simulink model "Grading_system"  (R2021a)
settings: Solver=VariableStepAuto  StartTime=0.0  StopTime=10.0  RelTol=1e-3
settings Model: Creator=Nour  LastModifiedBy=Nour

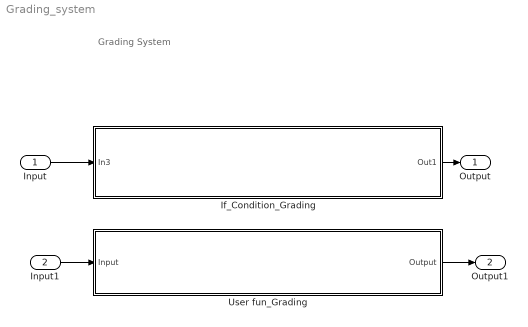
== system Grading_system ==
  note: Grading System
  Input : Inport
  Input1 : Inport  Port=2  OutDataTypeStr=uint8
  If_Condition_Grading : Subsystem
  User fun_Grading : Subsystem
  Output : Outport
  Output1 : Outport  Port=2
  wires:
  Input/1 -> If_Condition_Grading/1(In3)
  If_Condition_Grading/1(Out1) -> Output/1
  User fun_Grading/1(Output) -> Output1/1
  Input1/1 -> User fun_Grading/1(Input)

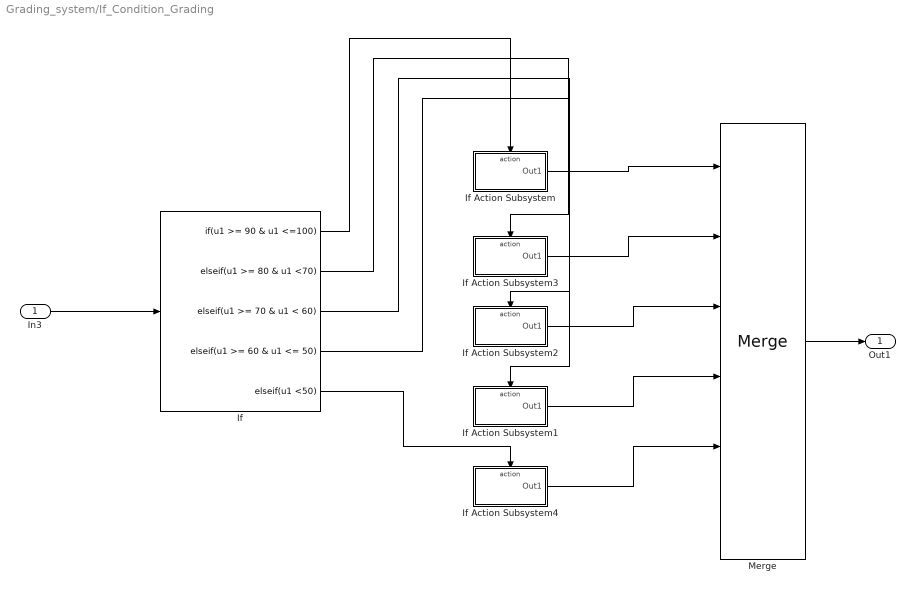
== system Grading_system/If_Condition_Grading ==
  In3 : Inport  OutDataTypeStr=uint8
  If : If  IfExpression=u1 >= 90 & u1 <=100  ElseIfExpressions=u1 >= 80 & u1 <70 , u1 >= 70 & u1 < 60, u1 >= 60 & u1 <= 50,u1 <50  ShowElse=off
  If Action Subsystem : Subsystem  TreatAsAtomicUnit=on
  If Action Subsystem1 : Subsystem  TreatAsAtomicUnit=on
  If Action Subsystem2 : Subsystem  TreatAsAtomicUnit=on
  If Action Subsystem3 : Subsystem  TreatAsAtomicUnit=on
  If Action Subsystem4 : Subsystem  TreatAsAtomicUnit=on
  Merge : Merge  Inputs=6
  Out1 : Outport
  wires:
  If Action Subsystem1/1(Out1) -> Merge/4
  If/4 -> If Action Subsystem1/Action
  If/3 -> If Action Subsystem2/Action
  If Action Subsystem4/1(Out1) -> Merge/5
  If/1 -> If Action Subsystem/Action
  If Action Subsystem2/1(Out1) -> Merge/3
  If/5 -> If Action Subsystem4/Action
  If/2 -> If Action Subsystem3/Action
  If Action Subsystem3/1(Out1) -> Merge/2
  If Action Subsystem/1(Out1) -> Merge/1
  In3/1 -> If/1
  Merge/1 -> Out1/1

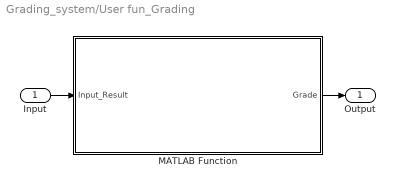
== system Grading_system/User fun_Grading ==
  Input : Inport  OutDataTypeStr=uint8
  MATLAB Function : MATLAB Function  TreatAsAtomicUnit=on
  Output : Outport  OutDataTypeStr=uint8
  wires:
  MATLAB Function/1(Grade) -> Output/1
  Input/1 -> MATLAB Function/1(Input_Result)

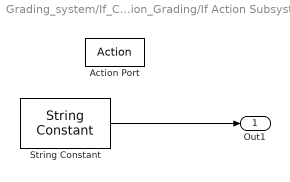
== system Grading_system/If_Condition_Grading/If Action Subsystem ==
  Action Port : ActionPort  ActionPortLabel=if(u1 >= 90 & u1 <=100)
  String Constant : StringConstant  String="\"A\""
  Out1 : Outport
  wires:
  String Constant/1 -> Out1/1

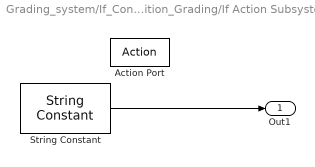
== system Grading_system/If_Condition_Grading/If Action Subsystem1 ==
  Action Port : ActionPort  ActionPortLabel=elseif( u1 >= 60 & u1 <= 50)
  String Constant : StringConstant  String="\"D\""
  Out1 : Outport
  wires:
  String Constant/1 -> Out1/1

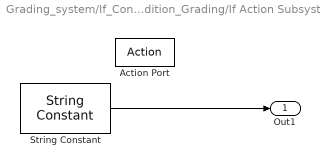
== system Grading_system/If_Condition_Grading/If Action Subsystem2 ==
  Action Port : ActionPort  ActionPortLabel=elseif( u1 >= 70 & u1 < 60)
  String Constant : StringConstant  String="\"C\""
  Out1 : Outport
  wires:
  String Constant/1 -> Out1/1

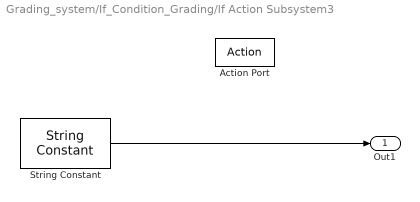
== system Grading_system/If_Condition_Grading/If Action Subsystem3 ==
  Action Port : ActionPort  ActionPortLabel=elseif(u1 >= 80 & u1 <70 )
  String Constant : StringConstant  String="\"B\""
  Out1 : Outport
  wires:
  String Constant/1 -> Out1/1

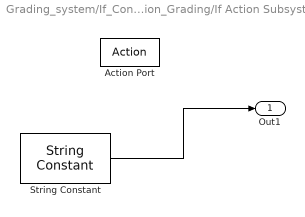
== system Grading_system/If_Condition_Grading/If Action Subsystem4 ==
  Action Port : ActionPort  ActionPortLabel=elseif(u1 <50)
  String Constant : StringConstant  String="\"F\""
  Out1 : Outport
  wires:
  String Constant/1 -> Out1/1

== matlab function Grading_system/User fun_Grading/MATLAB Function ==
  data: Input_Result input; Grade output
function Grade = fcn(Input_Result)

     if (score < 0 || score > 100)
        error("Invalid Result");
     end
     if (Input_Result >=90 && Input_Result <=100)
        Grade = 'A' ;
     elseif (Input_Result >=80 && Input_Result < 90)
         Grade = 'B' ;
     elseif (Input_Result >=70 && Input_Result < 80)
        Grade = 'C' ;
     elseif (Input_Result >= 60 && Input_Result < 70)
        Grade = 'D' ;
     else 
     Grade = 'F' ;
     end
        
     end
